simulink model "Smallestin4_Model"  (R2023a)
settings: Solver=VariableStepAuto  StartTime=0.0  StopTime=10.0  RelTol=1e-3
libraries: NSA_DEVS_SINKS_ATOMIC x5, NSA_DEVS_SOURCES_ATOMIC x4, NSA_DEVS_ROUTING_ATOMIC x1, NSA_DEVS_LOGISTICS_ATOMIC x1
settings Model: Creator=david  LastModifiedBy=david

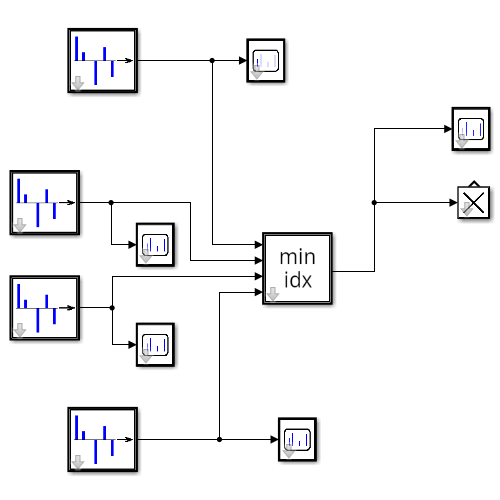
[thumbnail: Simulink's stored preview of the top-level diagram]
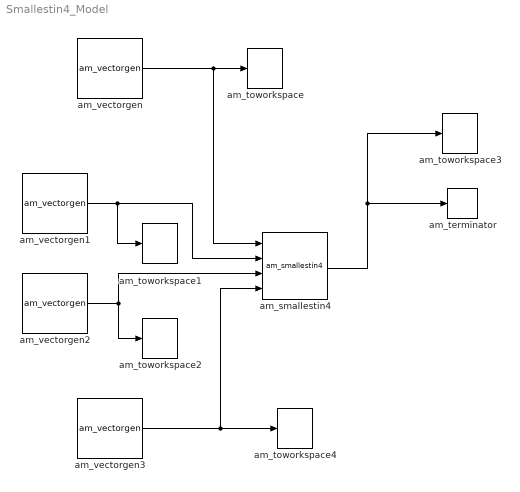
== system Smallestin4_Model ==
  am_smallestin4 : NSA_DEVS_ROUTING_ATOMIC/am_smallestin4  val0=0  tau=[0,1]  debug=0
      settings: SourceProductName=NSA_DEVS
  am_terminator : NSA_DEVS_LOGISTICS_ATOMIC/am_terminator  tau=[0,1]  debug=0
      settings: SourceProductName=NSA_DEVS
  am_toworkspace : NSA_DEVS_SINKS_ATOMIC/am_toworkspace  varname="\"gen1Out\""  t0=0  format="\"vector\""  tau=[0,5]  debug=0
      settings: SourceProductName=NSA_DEVS
  am_toworkspace1 : NSA_DEVS_SINKS_ATOMIC/am_toworkspace  varname="\"gen2Out\""  t0=0  format="\"vector\""  tau=[0,5]  debug=0
      settings: SourceProductName=NSA_DEVS
  am_toworkspace2 : NSA_DEVS_SINKS_ATOMIC/am_toworkspace  varname="\"gen3Out\""  t0=0  format="\"vector\""  tau=[0,5]  debug=0
      settings: SourceProductName=NSA_DEVS
  am_toworkspace3 : NSA_DEVS_SINKS_ATOMIC/am_toworkspace  varname="\"smallOut\""  t0=0  format="\"vector\""  tau=[0,5]  debug=0
      settings: SourceProductName=NSA_DEVS
  am_toworkspace4 : NSA_DEVS_SINKS_ATOMIC/am_toworkspace  varname="\"gen4Out\""  t0=0  format="\"vector\""  tau=[0,5]  debug=0
      settings: SourceProductName=NSA_DEVS
  am_vectorgen : NSA_DEVS_SOURCES_ATOMIC/am_vectorgen  tvec=[1, 3, 5, 7, 9]  yvec=[2, 3, 2, 5, 7]  tau=[0,1]  debug=0
      settings: SourceProductName=NSA_DEVS
  am_vectorgen1 : NSA_DEVS_SOURCES_ATOMIC/am_vectorgen  tvec=[1, 3, 5, 7.3, 9.3]  yvec=[1, 2, 3, 6, 7]  tau=[0,1]  debug=0
      settings: SourceProductName=NSA_DEVS
  am_vectorgen2 : NSA_DEVS_SOURCES_ATOMIC/am_vectorgen  tvec=[1, 3, 5, 7.6, 9.6]  yvec=[3, 1, 4, 7, 5]  tau=[0,1]  debug=0
      settings: SourceProductName=NSA_DEVS
  am_vectorgen3 : NSA_DEVS_SOURCES_ATOMIC/am_vectorgen  tvec=[1, 3, 5, 7.6, 9.6]  yvec=[0, 10, 1, 7, 5]  tau=[0,1]  debug=0
      settings: SourceProductName=NSA_DEVS
  wires:
  am_vectorgen1/1 -> am_smallestin4/2, am_toworkspace1/1
  am_vectorgen2/1 -> am_smallestin4/3, am_toworkspace2/1
  am_vectorgen/1 -> am_smallestin4/1, am_toworkspace/1
  am_smallestin4/1 -> am_toworkspace3/1, am_terminator/1
  am_vectorgen3/1 -> am_toworkspace4/1, am_smallestin4/4
